simulink model "transf2"  (R2022b)
settings: Solver=VariableStepAuto  StartTime=0.0  StopTime=10.0  RelTol=1e-3
values from neighbouring files (symbols this model uses):
  N = 3    [scriptLista3.m]
  Td = Kd/Kp    (= 0.133333333333)    [scriptLista3.m]
settings Model: Creator=vfton  LastModifiedBy=matak
settings ModelReferenceCC: EnableRefExpFcnMdlSchedulingChecks=on

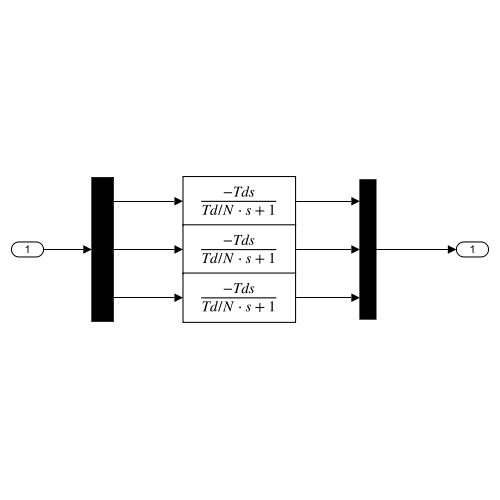
[thumbnail: Simulink's stored preview of the top-level diagram]
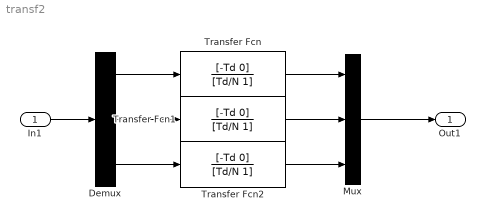
== system transf2 ==
  In1 : Inport
  Demux : Demux  Outputs=3
  Mux : Mux  Inputs=3
  Transfer Fcn : TransferFcn  Numerator=[-Td 0]  Denominator=[Td/N 1]
  Transfer Fcn1 : TransferFcn  Numerator=[-Td 0]  Denominator=[Td/N 1]
  Transfer Fcn2 : TransferFcn  Numerator=[-Td 0]  Denominator=[Td/N 1]
  Out1 : Outport
  wires:
  Demux/2 -> Transfer Fcn1/1
  Demux/3 -> Transfer Fcn2/1
  In1/1 -> Demux/1
  Transfer Fcn/1 -> Mux/1
  Demux/1 -> Transfer Fcn/1
  Transfer Fcn2/1 -> Mux/3
  Transfer Fcn1/1 -> Mux/2
  Mux/1 -> Out1/1
